simulink model "PubIfDecisionLM_MDL"  (R2020b)
settings: configuration reference "DspaceConfig" (kept outside this file)
PostLoadFcn:
  | if any(exist('dsrtsu_mdlpostloadfcn', 'file') ~= 0), dsrtsu_mdlpostloadfcn('Execute', bdroot); end
InitFcn:
  | , if any(exist('dsmpb_private', 'file') ~= 0), dsmpb_private('dsmpb_mdlclblib', 'Init', bdroot); end,
undefined symbols (not defined in the file or in its folder): OFM_OBJ_FUSIONTYPE_E, OFM_OBJ_MOVINGSTATE_E, OFM_OBJ_ORIENTATION_E, OFM_OBJ_TYPE_E, P_LM_Cyc, P_LM_EMLHistKapRcdBufSize, P_LM_EMLHistTrajBaseDis, P_LM_EMLHistTrajPNum, P_LM_EMLKapCorrMaxThre, P_LM_EMLMinKapThre, P_LM_EMLPathDisDiffThre, P_LM_EMLQuaFiltPar, P_LM_EMLTurnActKapThre, P_LM_EMLValidQuaThre, P_LM_FntPath1Disgap, P_LM_FntPath1MinDis, P_LM_FntPath1Timegap, P_LM_FntPath2Disgap, P_LM_FntPath2MinDis, P_LM_FntPath2Timegap, P_LM_FntPath3Disgap, P_LM_FntPath3MinDis, P_LM_FntPath3Timegap, P_LM_FusBLParFiltP, P_LM_FusEVDifC2Thre, P_LM_FusEVOPath1AllVSLDisThre, P_LM_FusEVOPath1AllVSLLostNumThre, P_LM_FusEVOPath1AllVSLQuaThre, P_LM_FusEVOPath1OTLFacNLC, P_LM_FusOTLQuaThre, P_LM_FusOTLSW, P_LM_FusParC0Index, P_LM_FusParC1Index, P_LM_FusParC2Index, P_LM_FusParC3Index, P_LM_FusVSLQuaThre, P_LM_FusVSLSW, P_LM_FusVSLValidSteerWheerAngThre, P_LM_FusVSLValidVxvThre, P_LM_LaneWidth, P_LM_OTLBufTPInfoEvaFactor, P_LM_OTLObjNum, P_LM_OTLObjSelectAgeThre, P_LM_OTLObjSelectDxAssessVx, P_LM_OTLObjSelectDxThre, P_LM_OTLObjSelectVxThre, P_LM_OTLObjSelectVyAssessDx, P_LM_OTLObjSelectVyThre, P_LM_OTLTrajPntBaseDis, P_LM_OTLTrajStdThre, P_LM_VSLAvailLineNum, P_LM_VSLBLSDiffThre, P_LM_VSLBLSDisRatio, P_LM_VSLFusBLParFiltP_C1, P_LM_VSLFusBLParFiltP_C2, P_LM_VSLFusBLParFiltP_C3, P_LM_VSLFusBLParFiltP_Quality, P_LM_VSLHistTrajBaseDis, P_LM_VSLHistTrajPNum, P_LM_VSLLCC0diff ... (+18)
libraries: simulink x145, LM_LIB x43
(part 20 of 24)

== matlab function PubIfDecisionLM_MDL/Subsystem2/LM_OTL/LM_OTL_MovObjTrajFit/LM_OTL_BufTPAssess/LM_OTL_BufTPInfoEva/MATLAB Function ==
  data: LM_OTLBufL1DxVect input; LM_OTLBufL2DxVect input; LM_OTLBufE1DxVect input; LM_OTLBufE2DxVect input; LM_OTLBufR1DxVect input; LM_OTLBufR2DxVect input; LM_OTLBufSPPosInfo input; LM_OTLBufEPPosInfo input; LM_OTLBufLastSPPosInfo input; LM_OTLBufLastEPPosInfo input; LM_FntPath1Dis input; LM_FntPath2Dis input; LM_FntPath3Dis input; LM_OTLBufL1LastValidInfo output; LM_OTLBufL2LastValidInfo output; LM_OTLBufE1LastValidInfo output; LM_OTLBufE2LastValidInfo output; LM_OTLBufR1LastValidInfo output; LM_OTLBufR2LastValidInfo output; LM_OTLBufL1ValidInfo output; LM_OTLBufL2ValidInfo output; LM_OTLBufE1ValidInfo output; LM_OTLBufE2ValidInfo output; LM_OTLBufR1ValidInfo output; LM_OTLBufR2ValidInfo output; P_LM_OTLBufTPInfoEvaFactor input
function [LM_OTLBufL1LastValidInfo,LM_OTLBufL2LastValidInfo,LM_OTLBufE1LastValidInfo,LM_OTLBufE2LastValidInfo,LM_OTLBufR1LastValidInfo,LM_OTLBufR2LastValidInfo,LM_OTLBufL1ValidInfo,LM_OTLBufL2ValidInfo,LM_OTLBufE1ValidInfo,LM_OTLBufE2ValidInfo,LM_OTLBufR1ValidInfo,LM_OTLBufR2ValidInfo] =fcn(LM_OTLBufL1DxVect,LM_OTLBufL2DxVect,LM_OTLBufE1DxVect,LM_OTLBufE2DxVect,LM_OTLBufR1DxVect,LM_OTLBufR2DxVect,LM_OTLBufSPPosInfo,LM_OTLBufEPPosInfo,LM_OTLBufLastSPPosInfo,LM_OTLBufLastEPPosInfo,LM_FntPath1Dis,LM_FntPath2Dis,LM_FntPath3Dis,P_LM_OTLBufTPInfoEvaFactor)

%%初始化基本参数
LM_OTLBufL1LastValidInfo=uint8(zeros(3,1));
LM_OTLBufL2LastValidInfo=uint8(zeros(3,1));
LM_OTLBufE1LastValidInfo=uint8(zeros(3,1));
LM_OTLBufE2LastValidInfo=uint8(zeros(3,1));
LM_OTLBufR1LastValidInfo=uint8(zeros(3,1));
LM_OTLBufR2LastValidInfo=uint8(zeros(3,1));
LM_OTLBufL1ValidInfo=uint8(zeros(3,1));
LM_OTLBufL2ValidInfo=uint8(zeros(3,1));
LM_OTLBufE1ValidInfo=uint8(zeros(3,1));
LM_OTLBufE2ValidInfo=uint8(zeros(3,1));
LM_OTLBufR1ValidInfo=uint8(zeros(3,1));
LM_OTLBufR2ValidInfo=uint8(zeros(3,1));
LM_FntPath0Dis=single(0);
%%计算车道线有效长度计算
FntPath1Length=LM_FntPath1Dis;
FntPath2Length=LM_FntPath2Dis-LM_FntPath1Dis;
FntPath3Length=LM_FntPath3Dis-LM_FntPath2Dis;
%%判断BufL1中前目标在各段车道线的有效值
if LM_OTLBufLastSPPosInfo(1)~=0
    %判断BufL1中前目标在前方第1段车道线的有效值
    t_buffer=[LM_OTLBufL1DxVect(LM_OTLBufLastSPPosInfo(1)),LM_OTLBufL1DxVect(LM_OTLBufLastEPPosInfo(1)),LM_FntPath0Dis,LM_FntPath1Dis];
    t_LMlength=abs(LM_OTLBufL1DxVect(LM_OTLBufLastSPPosInfo(1))-LM_OTLBufL1DxVect(LM_OTLBufLastEPPosInfo(1)));
    t_length=max(t_buffer)-min(t_buffer);
    t_overlap=FntPath1Length+t_LMlength-t_length;
    if t_overlap<P_LM_OTLBufTPInfoEvaFactor*FntPath1Length
        LM_OTLBufL1LastFntPath1Valid=0;
    else
        LM_OTLBufL1LastFntPath1Valid=1;
    end
    %判断BufL1中前目标在前方第2段车道线的有效值
    t_buffer=[LM_OTLBufL1DxVect(LM_OTLBufLastSPPosInfo(1)),LM_OTLBufL1DxVect(LM_OTLBufLastEPPosInfo(1)),LM_FntPath2Dis,LM_FntPath1Dis];
    t_length=max(t_buffer)-min(t_buffer);
    t_overlap=FntPath2Length+t_LMlength-t_length;
    if t_overlap<P_LM_OTLBufTPInfoEvaFactor*FntPath2Length
        LM_OTLBufL1LastFntPath2Valid=0;
    else
        LM_OTLBufL1LastFntPath2Valid=1;
    end
    %判断BufL1中前目标在前方第3段车道线的有效值
    t_buffer=[LM_OTLBufL1DxVect(LM_OTLBufLastSPPosInfo(1)),LM_OTLBufL1DxVect(LM_OTLBufLastEPPosInfo(1)),LM_FntPath2Dis,LM_FntPath3Dis];
    t_length=max(t_buffer)-min(t_buffer);
    t_overlap=FntPath3Length+t_LMlength-t_length;
    if t_overlap<P_LM_OTLBufTPInfoEvaFactor*FntPath3Length
        LM_OTLBufL1LastFntPath3Valid=0;
    else
        LM_OTLBufL1LastFntPath3Valid=1;
    end 
else
    LM_OTLBufL1LastFntPath1Valid=0;
    LM_OTLBufL1LastFntPath2Valid=0;
    LM_OTLBufL1LastFntPath3Valid=0;
end
LM_OTLBufL1LastValidInfo(1)=LM_OTLBufL1LastFntPath1Valid;
LM_OTLBufL1LastValidInfo(2)=LM_OTLBufL1LastFntPath2Valid;
LM_OTLBufL1LastValidInfo(3)=LM_OTLBufL1LastFntPath3Valid;
%%判断BufL1当前目标在各段车道线的有效值
if LM_OTLBufSPPosInfo(1)~=0
    %判断BufL1当前目标在前方第1段车道线的有效值
    t_LMlength=abs(LM_OTLBufL1DxVect(LM_OTLBufSPPosInfo(1))-LM_OTLBufL1DxVect(LM_OTLBufEPPosInfo(1)));
    t_buffer=[LM_OTLBufL1DxVect(LM_OTLBufSPPosInfo(1)),LM_OTLBufL1DxVect(LM_OTLBufEPPosInfo(1)),LM_FntPath0Dis,LM_FntPath1Dis];
    t_length=max(t_buffer)-min(t_buffer);
    t_overlap=FntPath1Length+t_LMlength-t_length;
    if t_overlap<P_LM_OTLBufTPInfoEvaFactor*FntPath1Length
        LM_OTLBufL1FntPath1Valid=0;
    else
        LM_OTLBufL1FntPath1Valid=1;
    end
    %判断BufL1当前目标在前方第2段车道线的有效值
    t_buffer=[LM_OTLBufL1DxVect(LM_OTLBufSPPosInfo(1)),LM_OTLBufL1DxVect(LM_OTLBufEPPosInfo(1)),LM_FntPath2Dis,LM_FntPath1Dis];
    t_length=max(t_buffer)-min(t_buffer);
    t_overlap=FntPath2Length+t_LMlength-t_length;
    if t_overlap<P_LM_OTLBufTPInfoEvaFactor*FntPath2Length
        LM_OTLBufL1FntPath2Valid=0;
    else
        LM_OTLBufL1FntPath2Valid=1;
    end
    %判断BufL1当前目标在前方第3段车道线的有效值
    t_buffer=[LM_OTLBufL1DxVect(LM_OTLBufSPPosInfo(1)),LM_OTLBufL1DxVect(LM_OTLBufEPPosInfo(1)),LM_FntPath2Dis,LM_FntPath3Dis];
    t_length=max(t_buffer)-min(t_buffer);
    t_overlap=FntPath3Length+t_LMlength-t_length;
    if t_overlap<P_LM_OTLBufTPInfoEvaFactor*FntPath3Length
        LM_OTLBufL1FntPath3Valid=0;
    else
        LM_OTLBufL1FntPath3Valid=1;
    end 
else
    LM_OTLBufL1FntPath1Valid=0;
    LM_OTLBufL1FntPath2Valid=0;
    LM_OTLBufL1FntPath3Valid=0;
end
LM_OTLBufL1ValidInfo(1)=LM_OTLBufL1FntPath1Valid;
LM_OTLBufL1ValidInfo(2)=LM_OTLBufL1FntPath2Valid;
LM_OTLBufL1ValidInfo(3)=LM_OTLBufL1FntPath3Valid;
%%判断BufL2中前目标在各段车道线的有效值
if LM_OTLBufLastSPPosInfo(2)~=0
    %判断BufL2中前目标在前方第1段车道线的有效值
    t_LMlength=abs(LM_OTLBufL2DxVect(LM_OTLBufLastSPPosInfo(2))-LM_OTLBufL2DxVect(LM_OTLBufLastEPPosInfo(2)));
    t_buffer=[LM_OTLBufL2DxVect(LM_OTLBufLastSPPosInfo(2)),LM_OTLBufL2DxVect(LM_OTLBufLastEPPosInfo(2)),LM_FntPath0Dis,LM_FntPath1Dis];
    t_length=max(t_buffer)-min(t_buffer);
    t_overlap=FntPath1Length+t_LMlength-t_length;
    if t_overlap<P_LM_OTLBufTPInfoEvaFactor*FntPath1Length
        LM_OTLBufL2LastFntPath1Valid=0;
    else
        LM_OTLBufL2LastFntPath1Valid=1;
    end
    %判断BufL2中前目标在前方第2段车道线的有效值
    t_buffer=[LM_OTLBufL2DxVect(LM_OTLBufLastSPPosInfo(2)),LM_OTLBufL2DxVect(LM_OTLBufLastEPPosInfo(2)),LM_FntPath2Dis,LM_FntPath1Dis];
    t_length=max(t_buffer)-min(t_buffer);
    t_overlap=FntPath2Length+t_LMlength-t_length;
    if t_overlap<P_LM_OTLBufTPInfoEvaFactor*FntPath2Length
        LM_OTLBufL2LastFntPath2Valid=0;
    else
        LM_OTLBufL2LastFntPath2Valid=1;
    end
    %判断BufL2中前目标在前方第3段车道线的有效值
    t_buffer=[LM_OTLBufL2DxVect(LM_OTLBufLastSPPosInfo(2)),LM_OTLBufL2DxVect(LM_OTLBufLastEPPosInfo(2)),LM_FntPath2Dis,LM_FntPath3Dis];
    t_length=max(t_buffer)-min(t_buffer);
    t_overlap=FntPath3Length+t_LMlength-t_length;
    if t_overlap<P_LM_OTLBufTPInfoEvaFactor*FntPath3Length
        LM_OTLBufL2LastFntPath3Valid=0;
    else
        LM_OTLBufL2LastFntPath3Valid=1;
    end 
else
    LM_OTLBufL2LastFntPath1Valid=0;
    LM_OTLBufL2LastFntPath2Valid=0;
    LM_OTLBufL2LastFntPath3Valid=0;
end
LM_OTLBufL2LastValidInfo(1)=LM_OTLBufL2LastFntPath1Valid;
LM_OTLBufL2LastValidInfo(2)=LM_OTLBufL2LastFntPath2Valid;
LM_OTLBufL2LastValidInfo(3)=LM_OTLBufL2LastFntPath3Valid;
%%判断BufL2当前目标在各段车道线的有效值
if LM_OTLBufSPPosInfo(2)~=0
    %判断BufL2当前目标在前方第1段车道线的有效值
    t_LMlength=abs(LM_OTLBufL2DxVect(LM_OTLBufSPPosInfo(2))-LM_OTLBufL2DxVect(LM_OTLBufEPPosInfo(2)));
    t_buffer=[LM_OTLBufL2DxVect(LM_OTLBufSPPosInfo(2)),LM_OTLBufL2DxVect(LM_OTLBufEPPosInfo(2)),LM_FntPath0Dis,LM_FntPath1Dis];
    t_length=max(t_buffer)-min(t_buffer);
    t_overlap=FntPath1Length+t_LMlength-t_length;
    if t_overlap<P_LM_OTLBufTPInfoEvaFactor*FntPath1Length
        LM_OTLBufL2FntPath1Valid=0;
    else
        LM_OTLBufL2FntPath1Valid=1;
    end
    %判断BufL2当前目标在前方第2段车道线的有效值
    t_buffer=[LM_OTLBufL2DxVect(LM_OTLBufSPPosInfo(2)),LM_OTLBufL2DxVect(LM_OTLBufEPPosInfo(2)),LM_FntPath2Dis,LM_FntPath1Dis];
    t_length=max(t_buffer)-min(t_buffer);
    t_overlap=FntPath2Length+t_LMlength-t_length;
    if t_overlap<P_LM_OTLBufTPInfoEvaFactor*FntPath2Length
        LM_OTLBufL2FntPath2Valid=0;
    else
        LM_OTLBufL2FntPath2Valid=1;
    end
    %判断BufL2当前目标在前方第3段车道线的有效值
    t_buffer=[LM_OTLBufL2DxVect(LM_OTLBufSPPosInfo(2)),LM_OTLBufL2DxVect(LM_OTLBufEPPosInfo(2)),LM_FntPath2Dis,LM_FntPath3Dis];
    t_length=max(t_buffer)-min(t_buffer);
    t_overlap=FntPath3Length+t_LMlength-t_length;
    if t_overlap<P_LM_OTLBufTPInfoEvaFactor*FntPath3Length
        LM_OTLBufL2FntPath3Valid=0;
    else
        LM_OTLBufL2FntPath3Valid=1;
    end 
else
    LM_OTLBufL2FntPath1Valid=0;
    LM_OTLBufL2FntPath2Valid=0;
    LM_OTLBufL2FntPath3Valid=0;
end
LM_OTLBufL2ValidInfo(1)=LM_OTLBufL2FntPath1Valid;
LM_OTLBufL2ValidInfo(2)=LM_OTLBufL2FntPath2Valid;
LM_OTLBufL2ValidInfo(3)=LM_OTLBufL2FntPath3Valid;
%%判断BufE1中前目标在各段车道线的有效值
if LM_OTLBufLastSPPosInfo(3)~=0
    %判断BufE1中前目标在前方第1段车道线的有效值
    t_LMlength=abs(LM_OTLBufE1DxVect(LM_OTLBufLastSPPosInfo(3))-LM_OTLBufE1DxVect(LM_OTLBufLastEPPosInfo(3)));
    t_buffer=[LM_OTLBufE1DxVect(LM_OTLBufLastSPPosInfo(3)),LM_OTLBufE1DxVect(LM_OTLBufLastEPPosInfo(3)),LM_FntPath0Dis,LM_FntPath1Dis];
    t_length=max(t_buffer)-min(t_buffer);
    t_overlap=FntPath1Length+t_LMlength-t_length;
    if t_overlap<P_LM_OTLBufTPInfoEvaFactor*FntPath1Length
        LM_OTLBufE1LastFntPath1Valid=0;
    else
        LM_OTLBufE1LastFntPath1Valid=1;
    end
    %判断BufE1中前目标在前方第2段车道线的有效值
    t_buffer=[LM_OTLBufE1DxVect(LM_OTLBufLastSPPosInfo(3)),LM_OTLBufE1DxVect(LM_OTLBufLastEPPosInfo(3)),LM_FntPath2Dis,LM_FntPath1Dis];
    t_length=max(t_buffer)-min(t_buffer);
    t_overlap=FntPath2Length+t_LMlength-t_length;
    if t_overlap<P_LM_OTLBufTPInfoEvaFactor*FntPath2Length
        LM_OTLBufE1LastFntPath2Valid=0;
    else
        LM_OTLBufE1LastFntPath2Valid=1;
    end
    %判断BufE1中前目标在前方第3段车道线的有效值
    t_buffer=[LM_OTLBufE1DxVect(LM_OTLBufLastSPPosInfo(3)),LM_OTLBufE1DxVect(LM_OTLBufLastEPPosInfo(3)),LM_FntPath2Dis,LM_FntPath3Dis];
    t_length=max(t_buffer)-min(t_buffer);
    t_overlap=FntPath3Length+t_LMlength-t_length;
    if t_overlap<P_LM_OTLBufTPInfoEvaFactor*FntPath3Length
        LM_OTLBufE1LastFntPath3Valid=0;
    else
        LM_OTLBufE1LastFntPath3Valid=1;
    end 
else
    LM_OTLBufE1LastFntPath1Valid=0;
    LM_OTLBufE1LastFntPath2Valid=0;
    LM_OTLBufE1LastFntPath3Valid=0;
end
LM_OTLBufE1LastValidInfo(1)=LM_OTLBufE1LastFntPath1Valid;
LM_OTLBufE1LastValidInfo(2)=LM_OTLBufE1LastFntPath2Valid;
LM_OTLBufE1LastValidInfo(3)=LM_OTLBufE1LastFntPath3Valid;
%%判断BufE1当前目标在各段车道线的有效值
if LM_OTLBufSPPosInfo(3)~=0
    %判断BufE1当前目标在前方第1段车道线的有效值
    t_LMlength=abs(LM_OTLBufE1DxVect(LM_OTLBufSPPosInfo(3))-LM_OTLBufE1DxVect(LM_OTLBufEPPosInfo(3)));
    t_buffer=[LM_OTLBufE1DxVect(LM_OTLBufSPPosInfo(3)),LM_OTLBufE1DxVect(LM_OTLBufEPPosInfo(3)),LM_FntPath0Dis,LM_FntPath1Dis];
    t_length=max(t_buffer)-min(t_buffer);
    t_overlap=FntPath1Length+t_LMlength-t_length;
    if t_overlap<P_LM_OTLBufTPInfoEvaFactor*FntPath1Length
        LM_OTLBufE1FntPath1Valid=0;
    else
        LM_OTLBufE1FntPath1Valid=1;
    end
    %判断BufE1当前目标在前方第2段车道线的有效值
    t_buffer=[LM_OTLBufE1DxVect(LM_OTLBufSPPosInfo(3)),LM_OTLBufE1DxVect(LM_OTLBufEPPosInfo(3)),LM_FntPath2Dis,LM_FntPath1Dis];
    t_length=max(t_buffer)-min(t_buffer);
    t_overlap=FntPath2Length+t_LMlength-t_length;
    if t_overlap<P_LM_OTLBufTPInfoEvaFactor*FntPath2Length
        LM_OTLBufE1FntPath2Valid=0;
    else
        LM_OTLBufE1FntPath2Valid=1;
    end
    %判断BufE1当前目标在前方第3段车道线的有效值
    t_buffer=[LM_OTLBufE1DxVect(LM_OTLBufSPPosInfo(3)),LM_OTLBufE1DxVect(LM_OTLBufEPPosInfo(3)),LM_FntPath2Dis,LM_FntPath3Dis];
    t_length=max(t_buffer)-min(t_buffer);
    t_overlap=FntPath3Length+t_LMlength-t_length;
    if t_overlap<P_LM_OTLBufTPInfoEvaFactor*FntPath3Length
        LM_OTLBufE1FntPath3Valid=0;
    else
        LM_OTLBufE1FntPath3Valid=1;
    end 
else
    LM_OTLBufE1FntPath1Valid=0;
    LM_OTLBufE1FntPath2Valid=0;
    LM_OTLBufE1FntPath3Valid=0;
end
LM_OTLBufE1ValidInfo(1)=LM_OTLBufE1FntPath1Valid;
LM_OTLBufE1ValidInfo(2)=LM_OTLBufE1FntPath2Valid;
LM_OTLBufE1ValidInfo(3)=LM_OTLBufE1FntPath3Valid;
%%判断BufE2中前目标在各段车道线的有效值
if LM_OTLBufLastSPPosInfo(4)~=0
    %判断BufE2中前目标在前方第1段车道线的有效值
    t_LMlength=abs(LM_OTLBufE2DxVect(LM_OTLBufLastSPPosInfo(4))-LM_OTLBufE2DxVect(LM_OTLBufLastEPPosInfo(4)));
    t_buffer=[LM_OTLBufE2DxVect(LM_OTLBufLastSPPosInfo(4)),LM_OTLBufE2DxVect(LM_OTLBufLastEPPosInfo(4)),LM_FntPath0Dis,LM_FntPath1Dis];
    t_length=max(t_buffer)-min(t_buffer);
    t_overlap=FntPath1Length+t_LMlength-t_length;
    if t_overlap<P_LM_OTLBufTPInfoEvaFactor*FntPath1Length
        LM_OTLBufE2LastFntPath1Valid=0;
    else
        LM_OTLBufE2LastFntPath1Valid=1;
    end
    %判断BufE2中前目标在前方第2段车道线的有效值
    t_buffer=[LM_OTLBufE2DxVect(LM_OTLBufLastSPPosInfo(4)),LM_OTLBufE2DxVect(LM_OTLBufLastEPPosInfo(4)),LM_FntPath2Dis,LM_FntPath1Dis];
    t_length=max(t_buffer)-min(t_buffer);
    t_overlap=FntPath2Length+t_LMlength-t_length;
    if t_overlap<P_LM_OTLBufTPInfoEvaFactor*FntPath2Length
        LM_OTLBufE2LastFntPath2Valid=0;
    else
        LM_OTLBufE2LastFntPath2Valid=1;
    end
    %判断BufE2中前目标在前方第3段车道线的有效值
    t_buffer=[LM_OTLBufE2DxVect(LM_OTLBufLastSPPosInfo(4)),LM_OTLBufE2DxVect(LM_OTLBufLastEPPosInfo(4)),LM_FntPath2Dis,LM_FntPath3Dis];
    t_length=max(t_buffer)-min(t_buffer);
    t_overlap=FntPath3Length+t_LMlength-t_length;
    if t_overlap<P_LM_OTLBufTPInfoEvaFactor*FntPath3Length
        LM_OTLBufE2LastFntPath3Valid=0;
    else
        LM_OTLBufE2LastFntPath3Valid=1;
    end 
else
    LM_OTLBufE2LastFntPath1Valid=0;
    LM_OTLBufE2LastFntPath2Valid=0;
    LM_OTLBufE2LastFntPath3Valid=0;
end
LM_OTLBufE2LastValidInfo(1)=LM_OTLBufE2LastFntPath1Valid;
LM_OTLBufE2LastValidInfo(2)=LM_OTLBufE2LastFntPath2Valid;
LM_OTLBufE2LastValidInfo(3)=LM_OTLBufE2LastFntPath3Valid;
%%判断BufE2当前目标在各段车道线的有效值
if LM_OTLBufSPPosInfo(4)~=0
    %判断BufE2当前目标在前方第1段车道线的有效值
    t_LMlength=abs(LM_OTLBufE2DxVect(LM_OTLBufSPPosInfo(4))-LM_OTLBufE2DxVect(LM_OTLBufEPPosInfo(4)));
    t_buffer=[LM_OTLBufE2DxVect(LM_OTLBufSPPosInfo(4)),LM_OTLBufE2DxVect(LM_OTLBufEPPosInfo(4)),LM_FntPath0Dis,LM_FntPath1Dis];
    t_length=max(t_buffer)-min(t_buffer);
    t_overlap=FntPath1Length+t_LMlength-t_length;
    if t_overlap<P_LM_OTLBufTPInfoEvaFactor*FntPath1Length
        LM_OTLBufE2FntPath1Valid=0;
    else
        LM_OTLBufE2FntPath1Valid=1;
    end
    %判断BufE2当前目标在前方第2段车道线的有效值
    t_buffer=[LM_OTLBufE2DxVect(LM_OTLBufSPPosInfo(4)),LM_OTLBufE2DxVect(LM_OTLBufEPPosInfo(4)),LM_FntPath2Dis,LM_FntPath1Dis];
    t_length=max(t_buffer)-min(t_buffer);
    t_overlap=FntPath2Length+t_LMlength-t_length;
    if t_overlap<P_LM_OTLBufTPInfoEvaFactor*FntPath2Length
        LM_OTLBufE2FntPath2Valid=0;
    else
        LM_OTLBufE2FntPath2Valid=1;
    end
    %判断BufE2当前目标在前方第3段车道线的有效值
    t_buffer=[LM_OTLBufE2DxVect(LM_OTLBufSPPosInfo(4)),LM_OTLBufE2DxVect(LM_OTLBufEPPosInfo(4)),LM_FntPath2Dis,LM_FntPath3Dis];
    t_length=max(t_buffer)-min(t_buffer);
    t_overlap=FntPath3Length+t_LMlength-t_length;
    if t_overlap<P_LM_OTLBufTPInfoEvaFactor*FntPath3Length
        LM_OTLBufE2FntPath3Valid=0;
    else
        LM_OTLBufE2FntPath3Valid=1;
    end 
else
    LM_OTLBufE2FntPath1Valid=0;
    LM_OTLBufE2FntPath2Valid=0;
    LM_OTLBufE2FntPath3Valid=0;
end
LM_OTLBufE2ValidInfo(1)=LM_OTLBufE2FntPath1Valid;
LM_OTLBufE2ValidInfo(2)=LM_OTLBufE2FntPath2Valid;
LM_OTLBufE2ValidInfo(3)=LM_OTLBufE2FntPath3Valid;
%%判断BufR1中前目标在各段车道线的有效值
if LM_OTLBufLastSPPosInfo(5)~=0
    %判断BufR1中前目标在前方第1段车道线的有效值
    t_LMlength=abs(LM_OTLBufR1DxVect(LM_OTLBufLastSPPosInfo(5))-LM_OTLBufR1DxVect(LM_OTLBufLastEPPosInfo(5)));
    t_buffer=[LM_OTLBufR1DxVect(LM_OTLBufLastSPPosInfo(5)),LM_OTLBufR1DxVect(LM_OTLBufLastEPPosInfo(5)),LM_FntPath0Dis,LM_FntPath1Dis];
    t_length=max(t_buffer)-min(t_buffer);
    t_overlap=FntPath1Length+t_LMlength-t_length;
    if t_overlap<P_LM_OTLBufTPInfoEvaFactor*FntPath1Length
        LM_OTLBufR1LastFntPath1Valid=0;
    else
        LM_OTLBufR1LastFntPath1Valid=1;
    end
    %判断BufR1中前目标在前方第2段车道线的有效值
    t_buffer=[LM_OTLBufR1DxVect(LM_OTLBufLastSPPosInfo(5)),LM_OTLBufR1DxVect(LM_OTLBufLastEPPosInfo(5)),LM_FntPath2Dis,LM_FntPath1Dis];
    t_length=max(t_buffer)-min(t_buffer);
    t_overlap=FntPath2Length+t_LMlength-t_length;
    if t_overlap<P_LM_OTLBufTPInfoEvaFactor*FntPath2Length
        LM_OTLBufR1LastFntPath2Valid=0;
    else
        LM_OTLBufR1LastFntPath2Valid=1;
    end
    %判断BufR1中前目标在前方第3段车道线的有效值
    t_buffer=[LM_OTLBufR1DxVect(LM_OTLBufLastSPPosInfo(5)),LM_OTLBufR1DxVect(LM_OTLBufLastEPPosInfo(5)),LM_FntPath2Dis,LM_FntPath3Dis];
    t_length=max(t_buffer)-min(t_buffer);
    t_overlap=FntPath3Length+t_LMlength-t_length;
    if t_overlap<P_LM_OTLBufTPInfoEvaFactor*FntPath3Length
        LM_OTLBufR1LastFntPath3Valid=0;
    else
        LM_OTLBufR1LastFntPath3Valid=1;
    end 
else
    LM_OTLBufR1LastFntPath1Valid=0;
    LM_OTLBufR1LastFntPath2Valid=0;
    LM_OTLBufR1LastFntPath3Valid=0;
end
LM_OTLBufR1LastValidInfo(1)=LM_OTLBufR1LastFntPath1Valid;
LM_OTLBufR1LastValidInfo(2)=LM_OTLBufR1LastFntPath2Valid;
LM_OTLBufR1LastValidInfo(3)=LM_OTLBufR1LastFntPath3Valid;
%%判断BufR1当前目标在各段车道线的有效值
if LM_OTLBufSPPosInfo(5)~=0
    %判断BufR1当前目标在前方第1段车道线的有效值
    t_LMlength=abs(LM_OTLBufR1DxVect(LM_OTLBufSPPosInfo(5))-LM_OTLBufR1DxVect(LM_OTLBufEPPosInfo(5)));
    t_buffer=[LM_OTLBufR1DxVect(LM_OTLBufSPPosInfo(5)),LM_OTLBufR1DxVect(LM_OTLBufEPPosInfo(5)),LM_FntPath0Dis,LM_FntPath1Dis];
    t_length=max(t_buffer)-min(t_buffer);
    t_overlap=FntPath1Length+t_LMlength-t_length;
    if t_overlap<P_LM_OTLBufTPInfoEvaFactor*FntPath1Length
        LM_OTLBufR1FntPath1Valid=0;
    else
        LM_OTLBufR1FntPath1Valid=1;
    end
    %判断BufR1当前目标在前方第2段车道线的有效值
    t_buffer=[LM_OTLBufR1DxVect(LM_OTLBufSPPosInfo(5)),LM_OTLBufR1DxVect(LM_OTLBufEPPosInfo(5)),LM_FntPath2Dis,LM_FntPath1Dis];
    t_length=max(t_buffer)-min(t_buffer);
    t_overlap=FntPath2Length+t_LMlength-t_length;
    if t_overlap<P_LM_OTLBufTPInfoEvaFactor*FntPath2Length
        LM_OTLBufR1FntPath2Valid=0;
    else
        LM_OTLBufR1FntPath2Valid=1;
    end
    %判断BufR1当前目标在前方第3段车道线的有效值
    t_buffer=[LM_OTLBufR1DxVect(LM_OTLBufSPPosInfo(5)),LM_OTLBufR1DxVect(LM_OTLBufEPPosInfo(5)),LM_FntPath2Dis,LM_FntPath3Dis];
    t_length=max(t_buffer)-min(t_buffer);
    t_overlap=FntPath3Length+t_LMlength-t_length;
    if t_overlap<P_LM_OTLBufTPInfoEvaFactor*FntPath3Length
        LM_OTLBufR1FntPath3Valid=0;
    else
        LM_OTLBufR1FntPath3Valid=1;
    end 
else
    LM_OTLBufR1FntPath1Valid=0;
    LM_OTLBufR1FntPath2Valid=0;
    LM_OTLBufR1FntPath3Valid=0;
end
LM_OTLBufR1ValidInfo(1)=LM_OTLBufR1FntPath1Valid;
LM_OTLBufR1ValidInfo(2)=LM_OTLBufR1FntPath2Valid;
LM_OTLBufR1ValidInfo(3)=LM_OTLBufR1FntPath3Valid;
%%判断BufR2中前目标在各段车道线的有效值
if LM_OTLBufLastSPPosInfo(6)~=0
    %判断BufR2中前目标在前方第1段车道线的有效值
    t_LMlength=abs(LM_OTLBufR2DxVect(LM_OTLBufLastSPPosInfo(6))-LM_OTLBufR2DxVect(LM_OTLBufLastEPPosInfo(6)));
    t_buffer=[LM_OTLBufR2DxVect(LM_OTLBufLastSPPosInfo(6)),LM_OTLBufR2DxVect(LM_OTLBufLastEPPosInfo(6)),LM_FntPath0Dis,LM_FntPath1Dis];
    t_length=max(t_buffer)-min(t_buffer);
    t_overlap=FntPath1Length+t_LMlength-t_length;
    if t_overlap<P_LM_OTLBufTPInfoEvaFactor*FntPath1Length
        LM_OTLBufR2LastFntPath1Valid=0;
    else
        LM_OTLBufR2LastFntPath1Valid=1;
    end
    %判断BufR2中前目标在前方第2段车道线的有效值
    t_buffer=[LM_OTLBufR2DxVect(LM_OTLBufLastSPPosInfo(6)),LM_OTLBufR2DxVect(LM_OTLBufLastEPPosInfo(6)),LM_FntPath2Dis,LM_FntPath1Dis];
    t_length=max(t_buffer)-min(t_buffer);
    t_overlap=FntPath2Length+t_LMlength-t_length;
    if t_overlap<P_LM_OTLBufTPInfoEvaFactor*FntPath2Length
        LM_OTLBufR2LastFntPath2Valid=0;
    else
        LM_OTLBufR2LastFntPath2Valid=1;
    end
    %判断BufR2中前目标在前方第3段车道线的有效值
    t_buffer=[LM_OTLBufR2DxVect(LM_OTLBufLastSPPosInfo(6)),LM_OTLBufR2DxVect(LM_OTLBufLastEPPosInfo(6)),LM_FntPath2Dis,LM_FntPath3Dis];
    t_length=max(t_buffer)-min(t_buffer);
    t_overlap=FntPath3Length+t_LMlength-t_length;
    if t_overlap<P_LM_OTLBufTPInfoEvaFactor*FntPath3Length
        LM_OTLBufR2LastFntPath3Valid=0;
    else
        LM_OTLBufR2LastFntPath3Valid=1;
    end 
else
    LM_OTLBufR2LastFntPath1Valid=0;
    LM_OTLBufR2LastFntPath2Valid=0;
    LM_OTLBufR2LastFntPath3Valid=0;
end
LM_OTLBufR2LastValidInfo(1)=LM_OTLBufR2LastFntPath1Valid;
LM_OTLBufR2LastValidInfo(2)=LM_OTLBufR2LastFntPath2Valid;
LM_OTLBufR2LastValidInfo(3)=LM_OTLBufR2LastFntPath3Valid;
%%判断BufR2当前目标在各段车道线的有效值
if LM_OTLBufSPPosInfo(6)~=0
    %判断BufR2当前目标在前方第1段车道线的有效值
    t_LMlength=abs(LM_OTLBufR2DxVect(LM_OTLBufSPPosInfo(6))-LM_OTLBufR2DxVect(LM_OTLBufEPPosInfo(6)));
    t_buffer=[LM_OTLBufR2DxVect(LM_OTLBufSPPosInfo(6)),LM_OTLBufR2DxVect(LM_OTLBufEPPosInfo(6)),LM_FntPath0Dis,LM_FntPath1Dis];
    t_length=max(t_buffer)-min(t_buffer);
    t_overlap=FntPath1Length+t_LMlength-t_length;
    if t_overlap<P_LM_OTLBufTPInfoEvaFactor*FntPath1Length
        LM_OTLBufR2FntPath1Valid=0;
    else
        LM_OTLBufR2FntPath1Valid=1;
    end
    %判断BufR2当前目标在前方第2段车道线的有效值
    t_buffer=[LM_OTLBufR2DxVect(LM_OTLBufSPPosInfo(6)),LM_OTLBufR2DxVect(LM_OTLBufEPPosInfo(6)),LM_FntPath2Dis,LM_FntPath1Dis];
    t_length=max(t_buffer)-min(t_buffer);
    t_overlap=FntPath2Length+t_LMlength-t_length;
    if t_overlap<P_LM_OTLBufTPInfoEvaFactor*FntPath2Length
        LM_OTLBufR2FntPath2Valid=0;
    else
        LM_OTLBufR2FntPath2Valid=1;
    end
    %判断BufR2当前目标在前方第3段车道线的有效值
    t_buffer=[LM_OTLBufR2DxVect(LM_OTLBufSPPosInfo(6)),LM_OTLBufR2DxVect(LM_OTLBufEPPosInfo(6)),LM_FntPath2Dis,LM_FntPath3Dis];
    t_length=max(t_buffer)-min(t_buffer);
    t_overlap=FntPath3Length+t_LMlength-t_length;
    if t_overlap<P_LM_OTLBufTPInfoEvaFactor*FntPath3Length
        LM_OTLBufR2FntPath3Valid=0;
    else
        LM_OTLBufR2FntPath3Valid=1;
    end 
else
    LM_OTLBufR2FntPath1Valid=0;
    LM_OTLBufR2FntPath2Valid=0;
    LM_OTLBufR2FntPath3Valid=0;
end
LM_OTLBufR2ValidInfo(1)=LM_OTLBufR2FntPath1Valid;
LM_OTLBufR2ValidInfo(2)=LM_OTLBufR2FntPath2Valid;
LM_OTLBufR2ValidInfo(3)=LM_OTLBufR2FntPath3Valid;
end

== matlab function PubIfDecisionLM_MDL/Subsystem2/LM_OTL/LM_OTL_MovObjTrajFit/LM_OTL_BufTPAssess/LM_OTL_BufTrajEva/Subsystem/MATLAB Function1 ==
  data: Offset output; Flg output; LM_OTLBufValidInfo input; LM_OTLDxVect input; LM_OTLDyVect input; LM_OTLSPPos input; LM_OTLEPPos input; LM_FntPath1Dis input; LM_FntPath2Dis input; LM_FntPath3Dis input; TpValidNum output; SPValidPos output; P_LM_OTLTrajStdThre input
function [Offset,Flg,TpValidNum,SPValidPos] = fcn(LM_OTLBufValidInfo,LM_OTLDxVect,LM_OTLDyVect,LM_OTLSPPos,LM_OTLEPPos,LM_FntPath1Dis,LM_FntPath2Dis,LM_FntPath3Dis, P_LM_OTLTrajStdThre)


%%第一段前车道线取点
Offset=single(zeros(3,1));
Flg=uint8(zeros(3,1));
TpValidNum=uint8(zeros(3,1));
SPValidPos=uint8(zeros(3,1));
t_pnum=uint8(0);
t_sumy=single(0);
t_sumerry=single(0);
t_index=uint8(0);
if LM_OTLBufValidInfo(1)~=0
    if LM_OTLEPPos>=LM_OTLSPPos
        for i=LM_OTLSPPos:LM_OTLEPPos
            if LM_OTLDxVect(i)>0&&LM_OTLDxVect(i)<=LM_FntPath1Dis
                t_pnum=t_pnum+uint8(1);
                t_index=i;
                t_sumy=t_sumy+LM_OTLDyVect(i);
            end
        end
        t_mean=t_sumy/single(t_pnum);
        SPValidPos(1)=t_index-t_pnum+uint8(1);
        for i=t_index:-1:SPValidPos(1)
            t_error=(LM_OTLDyVect(i)-t_mean)^2;
            t_sumerry=t_sumerry+t_error;
        end
        if sqrt(t_sumerry/single(t_pnum))<=P_LM_OTLTrajStdThre
           Offset(1)=t_mean;
           Flg(1)=uint8(1);
           TpValidNum(1)=t_pnum;
        end
    elseif LM_OTLEPPos<LM_OTLSPPos
        for i=LM_OTLSPPos:80
            if LM_OTLDxVect(i)>0&&LM_OTLDxVect(i)<=LM_FntPath1Dis
                t_pnum=t_pnum+uint8(1);
                t_index=i;
                t_sumy=t_sumy+LM_OTLDyVect(i);
            end
        end
        for i=1:LM_OTLEPPos 
            if LM_OTLDxVect(i)>0&&LM_OTLDxVect(i)<=LM_FntPath1Dis
                t_pnum=t_pnum+uint8(1);
                t_index=i;
                t_sumy=t_sumy+LM_OTLDyVect(i);
            end
        end
        SPValidPos(1)=uint8(81)+t_index-t_pnum;
        t_mean=t_sumy/single(t_pnum);
        if SPValidPos(1)>80
            SPValidPos(1)=SPValidPos(1)-80;
        end
        if (SPValidPos(1)>=LM_OTLSPPos&&t_index>=LM_OTLSPPos)||(SPValidPos(1)<LM_OTLSPPos&&t_index<LM_OTLSPPos)
            for i=t_index:-1:SPValidPos(1)
                t_error=(LM_OTLDyVect(i)-t_mean)^2;
                t_sumerry=t_sumerry+t_error;
            end
        else
            for i=1:t_index
                t_error=(LM_OTLDyVect(i)-t_mean)^2;
                t_sumerry=t_sumerry+t_error;
            end
            for i=80:-1:SPValidPos(1)
                 t_error=(LM_OTLDyVect(i)-t_mean)^2;
                t_sumerry=t_sumerry+t_error;
            end
        end
        if sqrt(t_sumerry/single(t_pnum))<=P_LM_OTLTrajStdThre
           Offset(1)=t_mean;
           Flg(1)=uint8(1);
           TpValidNum(1)=t_pnum;
        end           
    end
end
%%第二段前车道线取点
t_pnum=uint8(0);
t_sumy=single(0);
t_sumerry=single(0);
t_index=uint8(0);
if LM_OTLBufValidInfo(2)~=0
    if LM_OTLEPPos>=LM_OTLSPPos
        for i=LM_OTLSPPos:LM_OTLEPPos
            if LM_OTLDxVect(i)>LM_FntPath1Dis&&LM_OTLDxVect(i)<=LM_FntPath2Dis
                t_pnum=t_pnum+uint8(1);
                t_index=i;
                t_sumy=t_sumy+LM_OTLDyVect(i);
            end
        end
        t_mean=t_sumy/single(t_pnum);
        SPValidPos(2)=t_index-t_pnum+uint8(1);
        for i=t_index:-1:SPValidPos(2)
            t_error=(LM_OTLDyVect(i)-t_mean)^2;
            t_sumerry=t_sumerry+t_error;
        end
        if sqrt(t_sumerry/single(t_pnum))<=P_LM_OTLTrajStdThre
           Offset(2)=t_mean;
           Flg(2)=uint8(1);
           TpValidNum(2)=t_pnum;
        end
    elseif LM_OTLEPPos<LM_OTLSPPos
        for i=LM_OTLSPPos:80
            if LM_OTLDxVect(i)>LM_FntPath1Dis&&LM_OTLDxVect(i)<=LM_FntPath2Dis
                t_pnum=t_pnum+uint8(1);
                t_index=i;
                t_sumy=t_sumy+LM_OTLDyVect(i);
            end
        end
        for i=1:LM_OTLEPPos 
            if LM_OTLDxVect(i)>LM_FntPath1Dis&&LM_OTLDxVect(i)<=LM_FntPath2Dis
                t_pnum=t_pnum+uint8(1);
                t_index=i;
                t_sumy=t_sumy+LM_OTLDyVect(i);
            end
        end
        t_mean=t_sumy/single(t_pnum);
        SPValidPos(2)=uint8(81)+t_index-t_pnum;
        if SPValidPos(2)>80
            SPValidPos(2)=SPValidPos(2)-80;
        end
        if (SPValidPos(2)>=LM_OTLSPPos&&t_index>=LM_OTLSPPos)||(SPValidPos(2)<LM_OTLSPPos&&t_index<LM_OTLSPPos)
            for i=t_index:-1:SPValidPos(2)
                t_error=(LM_OTLDyVect(i)-t_mean)^2;
                t_sumerry=t_sumerry+t_error;
            end
        else
            for i=1:t_index
                t_error=(LM_OTLDyVect(i)-t_mean)^2;
                t_sumerry=t_sumerry+t_error;
            end
            for i=80:-1:SPValidPos(2)
                t_error=(LM_OTLDyVect(i)-t_mean)^2;
                t_sumerry=t_sumerry+t_error;
            end
        end
        if sqrt(t_sumerry/single(t_pnum))<=P_LM_OTLTrajStdThre
           Offset(2)=t_mean;
           Flg(2)=uint8(1);
           TpValidNum(2)=t_pnum;
        end           
    end
end
%%第三段前车道线取点
t_pnum=uint8(0);
t_sumy=single(0);
t_sumerry=single(0);
t_index=uint8(0);
if LM_OTLBufValidInfo(3)~=0
    if LM_OTLEPPos>=LM_OTLSPPos
        for i=LM_OTLSPPos:LM_OTLEPPos
            if LM_OTLDxVect(i)>LM_FntPath2Dis&&LM_OTLDxVect(i)<=LM_FntPath3Dis
                t_pnum=t_pnum+uint8(1);
                t_index=i;
                t_sumy=t_sumy+LM_OTLDyVect(i);
            end
        end
        SPValidPos(3)=t_index-t_pnum+1;
        t_mean=t_sumy/single(t_pnum);
        for i=t_index:-1:SPValidPos(3)
            t_error=(LM_OTLDyVect(i)-t_mean)^2;
            t_sumerry=t_sumerry+t_error;
        end
        if sqrt(t_sumerry/single(t_pnum))<=P_LM_OTLTrajStdThre
           Offset(3)=t_mean;
           Flg(3)=uint8(1);
           TpValidNum(3)=t_pnum;
        end
    elseif LM_OTLEPPos<LM_OTLSPPos
        for i=LM_OTLSPPos:80
            if LM_OTLDxVect(i)>LM_FntPath2Dis&&LM_OTLDxVect(i)<=LM_FntPath3Dis
                t_pnum=t_pnum+uint8(1);
                t_index=i;
                t_sumy=t_sumy+LM_OTLDyVect(i);
            end
        end
        for i=1:LM_OTLEPPos 
            if LM_OTLDxVect(i)>LM_FntPath2Dis&&LM_OTLDxVect(i)<=LM_FntPath3Dis
                t_pnum=t_pnum+uint8(1);
                t_index=i;
                t_sumy=t_sumy+LM_OTLDyVect(i);
            end
        end
        t_mean=t_sumy/single(t_pnum);
        SPValidPos(3)=uint8(81)+t_index-t_pnum;
        if SPValidPos(3)>80
            SPValidPos(3)=SPValidPos(3)-80;
        end
        if (SPValidPos(3)>=LM_OTLSPPos&&t_index>=LM_OTLSPPos)||(SPValidPos(3)<LM_OTLSPPos&&t_index<LM_OTLSPPos)
            for i=t_index:-1:SPValidPos(3)
                t_error=(LM_OTLDyVect(i)-t_mean)^2;
                t_sumerry=t_sumerry+t_error;
            end
        else
            for i=1:t_index
                t_error=(LM_OTLDyVect(i)-t_mean)^2;
                t_sumerry=t_sumerry+t_error;
            end
            for i=80:-1:SPValidPos(3)
                t_error=(LM_OTLDyVect(i)-t_mean)^2;
                t_sumerry=t_sumerry+t_error;
            end
        end
        if sqrt(t_sumerry/single(t_pnum))<=P_LM_OTLTrajStdThre
           Offset(3)=t_mean;
           Flg(3)=uint8(1);
           TpValidNum(3)=t_pnum;
        end           
    end
end
end

== matlab function PubIfDecisionLM_MDL/Subsystem2/LM_OTL/LM_OTL_MovObjTrajFit/LM_OTL_BufTPAssess/LM_OTL_BufTrajEva/Subsystem1/MATLAB Function1 ==
  data: Offset output; Flg output; LM_OTLBufValidInfo input; LM_OTLDxVect input; LM_OTLDyVect input; LM_OTLSPPos input; LM_OTLEPPos input; LM_FntPath1Dis input; LM_FntPath2Dis input; LM_FntPath3Dis input; TpValidNum output; SPValidPos output; P_LM_OTLTrajStdThre input
function [Offset,Flg,TpValidNum,SPValidPos] = fcn(LM_OTLBufValidInfo,LM_OTLDxVect,LM_OTLDyVect,LM_OTLSPPos,LM_OTLEPPos,LM_FntPath1Dis,LM_FntPath2Dis,LM_FntPath3Dis, P_LM_OTLTrajStdThre)


%%第一段前车道线取点
Offset=single(zeros(3,1));
Flg=uint8(zeros(3,1));
TpValidNum=uint8(zeros(3,1));
SPValidPos=uint8(zeros(3,1));
t_pnum=uint8(0);
t_sumy=single(0);
t_sumerry=single(0);
t_index=uint8(0);
if LM_OTLBufValidInfo(1)~=0
    if LM_OTLEPPos>=LM_OTLSPPos
        for i=LM_OTLSPPos:LM_OTLEPPos
            if LM_OTLDxVect(i)>0&&LM_OTLDxVect(i)<=LM_FntPath1Dis
                t_pnum=t_pnum+uint8(1);
                t_index=i;
                t_sumy=t_sumy+LM_OTLDyVect(i);
            end
        end
        t_mean=t_sumy/single(t_pnum);
        SPValidPos(1)=t_index-t_pnum+uint8(1);
        for i=t_index:-1:SPValidPos(1)
            t_error=(LM_OTLDyVect(i)-t_mean)^2;
            t_sumerry=t_sumerry+t_error;
        end
        if sqrt(t_sumerry/single(t_pnum))<=P_LM_OTLTrajStdThre
           Offset(1)=t_mean;
           Flg(1)=uint8(1);
           TpValidNum(1)=t_pnum;
        end
    elseif LM_OTLEPPos<LM_OTLSPPos
        for i=LM_OTLSPPos:80
            if LM_OTLDxVect(i)>0&&LM_OTLDxVect(i)<=LM_FntPath1Dis
                t_pnum=t_pnum+uint8(1);
                t_index=i;
                t_sumy=t_sumy+LM_OTLDyVect(i);
            end
        end
        for i=1:LM_OTLEPPos 
            if LM_OTLDxVect(i)>0&&LM_OTLDxVect(i)<=LM_FntPath1Dis
                t_pnum=t_pnum+uint8(1);
                t_index=i;
                t_sumy=t_sumy+LM_OTLDyVect(i);
            end
        end
        SPValidPos(1)=uint8(81)+t_index-t_pnum;
        t_mean=t_sumy/single(t_pnum);
        if SPValidPos(1)>80
            SPValidPos(1)=SPValidPos(1)-80;
        end
        if (SPValidPos(1)>=LM_OTLSPPos&&t_index>=LM_OTLSPPos)||(SPValidPos(1)<LM_OTLSPPos&&t_index<LM_OTLSPPos)
            for i=t_index:-1:SPValidPos(1)
                t_error=(LM_OTLDyVect(i)-t_mean)^2;
                t_sumerry=t_sumerry+t_error;
            end
        else
            for i=1:t_index
                t_error=(LM_OTLDyVect(i)-t_mean)^2;
                t_sumerry=t_sumerry+t_error;
            end
            for i=80:-1:SPValidPos(1)
                 t_error=(LM_OTLDyVect(i)-t_mean)^2;
                t_sumerry=t_sumerry+t_error;
            end
        end
        if sqrt(t_sumerry/single(t_pnum))<=P_LM_OTLTrajStdThre
           Offset(1)=t_mean;
           Flg(1)=uint8(1);
           TpValidNum(1)=t_pnum;
        end           
    end
end
%%第二段前车道线取点
t_pnum=uint8(0);
t_sumy=single(0);
t_sumerry=single(0);
t_index=uint8(0);
if LM_OTLBufValidInfo(2)~=0
    if LM_OTLEPPos>=LM_OTLSPPos
        for i=LM_OTLSPPos:LM_OTLEPPos
            if LM_OTLDxVect(i)>LM_FntPath1Dis&&LM_OTLDxVect(i)<=LM_FntPath2Dis
                t_pnum=t_pnum+uint8(1);
                t_index=i;
                t_sumy=t_sumy+LM_OTLDyVect(i);
            end
        end
        t_mean=t_sumy/single(t_pnum);
        SPValidPos(2)=t_index-t_pnum+uint8(1);
        for i=t_index:-1:SPValidPos(2)
            t_error=(LM_OTLDyVect(i)-t_mean)^2;
            t_sumerry=t_sumerry+t_error;
        end
        if sqrt(t_sumerry/single(t_pnum))<=P_LM_OTLTrajStdThre
           Offset(2)=t_mean;
           Flg(2)=uint8(1);
           TpValidNum(2)=t_pnum;
        end
    elseif LM_OTLEPPos<LM_OTLSPPos
        for i=LM_OTLSPPos:80
            if LM_OTLDxVect(i)>LM_FntPath1Dis&&LM_OTLDxVect(i)<=LM_FntPath2Dis
                t_pnum=t_pnum+uint8(1);
                t_index=i;
                t_sumy=t_sumy+LM_OTLDyVect(i);
            end
        end
        for i=1:LM_OTLEPPos 
            if LM_OTLDxVect(i)>LM_FntPath1Dis&&LM_OTLDxVect(i)<=LM_FntPath2Dis
                t_pnum=t_pnum+uint8(1);
                t_index=i;
                t_sumy=t_sumy+LM_OTLDyVect(i);
            end
        end
        t_mean=t_sumy/single(t_pnum);
        SPValidPos(2)=uint8(81)+t_index-t_pnum;
        if SPValidPos(2)>80
            SPValidPos(2)=SPValidPos(2)-80;
        end
        if (SPValidPos(2)>=LM_OTLSPPos&&t_index>=LM_OTLSPPos)||(SPValidPos(2)<LM_OTLSPPos&&t_index<LM_OTLSPPos)
            for i=t_index:-1:SPValidPos(2)
                t_error=(LM_OTLDyVect(i)-t_mean)^2;
                t_sumerry=t_sumerry+t_error;
            end
        else
            for i=1:t_index
                t_error=(LM_OTLDyVect(i)-t_mean)^2;
                t_sumerry=t_sumerry+t_error;
            end
            for i=80:-1:SPValidPos(2)
                t_error=(LM_OTLDyVect(i)-t_mean)^2;
                t_sumerry=t_sumerry+t_error;
            end
        end
        if sqrt(t_sumerry/single(t_pnum))<=P_LM_OTLTrajStdThre
           Offset(2)=t_mean;
           Flg(2)=uint8(1);
           TpValidNum(2)=t_pnum;
        end           
    end
end
%%第三段前车道线取点
t_pnum=uint8(0);
t_sumy=single(0);
t_sumerry=single(0);
t_index=uint8(0);
if LM_OTLBufValidInfo(3)~=0
    if LM_OTLEPPos>=LM_OTLSPPos
        for i=LM_OTLSPPos:LM_OTLEPPos
            if LM_OTLDxVect(i)>LM_FntPath2Dis&&LM_OTLDxVect(i)<=LM_FntPath3Dis
                t_pnum=t_pnum+uint8(1);
                t_index=i;
                t_sumy=t_sumy+LM_OTLDyVect(i);
            end
        end
        SPValidPos(3)=t_index-t_pnum+1;
        t_mean=t_sumy/single(t_pnum);
        for i=t_index:-1:SPValidPos(3)
            t_error=(LM_OTLDyVect(i)-t_mean)^2;
            t_sumerry=t_sumerry+t_error;
        end
        if sqrt(t_sumerry/single(t_pnum))<=P_LM_OTLTrajStdThre
           Offset(3)=t_mean;
           Flg(3)=uint8(1);
           TpValidNum(3)=t_pnum;
        end
    elseif LM_OTLEPPos<LM_OTLSPPos
        for i=LM_OTLSPPos:80
            if LM_OTLDxVect(i)>LM_FntPath2Dis&&LM_OTLDxVect(i)<=LM_FntPath3Dis
                t_pnum=t_pnum+uint8(1);
                t_index=i;
                t_sumy=t_sumy+LM_OTLDyVect(i);
            end
        end
        for i=1:LM_OTLEPPos 
            if LM_OTLDxVect(i)>LM_FntPath2Dis&&LM_OTLDxVect(i)<=LM_FntPath3Dis
                t_pnum=t_pnum+uint8(1);
                t_index=i;
                t_sumy=t_sumy+LM_OTLDyVect(i);
            end
        end
        t_mean=t_sumy/single(t_pnum);
        SPValidPos(3)=uint8(81)+t_index-t_pnum;
        if SPValidPos(3)>80
            SPValidPos(3)=SPValidPos(3)-80;
        end
        if (SPValidPos(3)>=LM_OTLSPPos&&t_index>=LM_OTLSPPos)||(SPValidPos(3)<LM_OTLSPPos&&t_index<LM_OTLSPPos)
            for i=t_index:-1:SPValidPos(3)
                t_error=(LM_OTLDyVect(i)-t_mean)^2;
                t_sumerry=t_sumerry+t_error;
            end
        else
            for i=1:t_index
                t_error=(LM_OTLDyVect(i)-t_mean)^2;
                t_sumerry=t_sumerry+t_error;
            end
            for i=80:-1:SPValidPos(3)
                t_error=(LM_OTLDyVect(i)-t_mean)^2;
                t_sumerry=t_sumerry+t_error;
            end
        end
        if sqrt(t_sumerry/single(t_pnum))<=P_LM_OTLTrajStdThre
           Offset(3)=t_mean;
           Flg(3)=uint8(1);
           TpValidNum(3)=t_pnum;
        end           
    end
end
end

== matlab function PubIfDecisionLM_MDL/Subsystem2/LM_OTL/LM_OTL_MovObjTrajFit/LM_OTL_BufTPAssess/LM_OTL_BufTrajEva/Subsystem10/MATLAB Function1 ==
  data: Offset output; Flg output; LM_OTLBufValidInfo input; LM_OTLDxVect input; LM_OTLDyVect input; LM_OTLSPPos input; LM_OTLEPPos input; LM_FntPath1Dis input; LM_FntPath2Dis input; LM_FntPath3Dis input; TpValidNum output; SPValidPos output; P_LM_OTLTrajStdThre input
function [Offset,Flg,TpValidNum,SPValidPos] = fcn(LM_OTLBufValidInfo,LM_OTLDxVect,LM_OTLDyVect,LM_OTLSPPos,LM_OTLEPPos,LM_FntPath1Dis,LM_FntPath2Dis,LM_FntPath3Dis, P_LM_OTLTrajStdThre)


%%第一段前车道线取点
Offset=single(zeros(3,1));
Flg=uint8(zeros(3,1));
TpValidNum=uint8(zeros(3,1));
SPValidPos=uint8(zeros(3,1));
t_pnum=uint8(0);
t_sumy=single(0);
t_sumerry=single(0);
t_index=uint8(0);
if LM_OTLBufValidInfo(1)~=0
    if LM_OTLEPPos>=LM_OTLSPPos
        for i=LM_OTLSPPos:LM_OTLEPPos
            if LM_OTLDxVect(i)>0&&LM_OTLDxVect(i)<=LM_FntPath1Dis
                t_pnum=t_pnum+uint8(1);
                t_index=i;
                t_sumy=t_sumy+LM_OTLDyVect(i);
            end
        end
        t_mean=t_sumy/single(t_pnum);
        SPValidPos(1)=t_index-t_pnum+uint8(1);
        for i=t_index:-1:SPValidPos(1)
            t_error=(LM_OTLDyVect(i)-t_mean)^2;
            t_sumerry=t_sumerry+t_error;
        end
        if sqrt(t_sumerry/single(t_pnum))<=P_LM_OTLTrajStdThre
           Offset(1)=t_mean;
           Flg(1)=uint8(1);
           TpValidNum(1)=t_pnum;
        end
    elseif LM_OTLEPPos<LM_OTLSPPos
        for i=LM_OTLSPPos:80
            if LM_OTLDxVect(i)>0&&LM_OTLDxVect(i)<=LM_FntPath1Dis
                t_pnum=t_pnum+uint8(1);
                t_index=i;
                t_sumy=t_sumy+LM_OTLDyVect(i);
            end
        end
        for i=1:LM_OTLEPPos 
            if LM_OTLDxVect(i)>0&&LM_OTLDxVect(i)<=LM_FntPath1Dis
                t_pnum=t_pnum+uint8(1);
                t_index=i;
                t_sumy=t_sumy+LM_OTLDyVect(i);
            end
        end
        SPValidPos(1)=uint8(81)+t_index-t_pnum;
        t_mean=t_sumy/single(t_pnum);
        if SPValidPos(1)>80
            SPValidPos(1)=SPValidPos(1)-80;
        end
        if (SPValidPos(1)>=LM_OTLSPPos&&t_index>=LM_OTLSPPos)||(SPValidPos(1)<LM_OTLSPPos&&t_index<LM_OTLSPPos)
            for i=t_index:-1:SPValidPos(1)
                t_error=(LM_OTLDyVect(i)-t_mean)^2;
                t_sumerry=t_sumerry+t_error;
            end
        else
            for i=1:t_index
                t_error=(LM_OTLDyVect(i)-t_mean)^2;
                t_sumerry=t_sumerry+t_error;
            end
            for i=80:-1:SPValidPos(1)
                 t_error=(LM_OTLDyVect(i)-t_mean)^2;
                t_sumerry=t_sumerry+t_error;
            end
        end
        if sqrt(t_sumerry/single(t_pnum))<=P_LM_OTLTrajStdThre
           Offset(1)=t_mean;
           Flg(1)=uint8(1);
           TpValidNum(1)=t_pnum;
        end           
    end
end
%%第二段前车道线取点
t_pnum=uint8(0);
t_sumy=single(0);
t_sumerry=single(0);
t_index=uint8(0);
if LM_OTLBufValidInfo(2)~=0
    if LM_OTLEPPos>=LM_OTLSPPos
        for i=LM_OTLSPPos:LM_OTLEPPos
            if LM_OTLDxVect(i)>LM_FntPath1Dis&&LM_OTLDxVect(i)<=LM_FntPath2Dis
                t_pnum=t_pnum+uint8(1);
                t_index=i;
                t_sumy=t_sumy+LM_OTLDyVect(i);
            end
        end
        t_mean=t_sumy/single(t_pnum);
        SPValidPos(2)=t_index-t_pnum+uint8(1);
        for i=t_index:-1:SPValidPos(2)
            t_error=(LM_OTLDyVect(i)-t_mean)^2;
            t_sumerry=t_sumerry+t_error;
        end
        if sqrt(t_sumerry/single(t_pnum))<=P_LM_OTLTrajStdThre
           Offset(2)=t_mean;
           Flg(2)=uint8(1);
           TpValidNum(2)=t_pnum;
        end
    elseif LM_OTLEPPos<LM_OTLSPPos
        for i=LM_OTLSPPos:80
            if LM_OTLDxVect(i)>LM_FntPath1Dis&&LM_OTLDxVect(i)<=LM_FntPath2Dis
                t_pnum=t_pnum+uint8(1);
                t_index=i;
                t_sumy=t_sumy+LM_OTLDyVect(i);
            end
        end
        for i=1:LM_OTLEPPos 
            if LM_OTLDxVect(i)>LM_FntPath1Dis&&LM_OTLDxVect(i)<=LM_FntPath2Dis
                t_pnum=t_pnum+uint8(1);
                t_index=i;
                t_sumy=t_sumy+LM_OTLDyVect(i);
            end
        end
        t_mean=t_sumy/single(t_pnum);
        SPValidPos(2)=uint8(81)+t_index-t_pnum;
        if SPValidPos(2)>80
            SPValidPos(2)=SPValidPos(2)-80;
        end
        if (SPValidPos(2)>=LM_OTLSPPos&&t_index>=LM_OTLSPPos)||(SPValidPos(2)<LM_OTLSPPos&&t_index<LM_OTLSPPos)
            for i=t_index:-1:SPValidPos(2)
                t_error=(LM_OTLDyVect(i)-t_mean)^2;
                t_sumerry=t_sumerry+t_error;
            end
        else
            for i=1:t_index
                t_error=(LM_OTLDyVect(i)-t_mean)^2;
                t_sumerry=t_sumerry+t_error;
            end
            for i=80:-1:SPValidPos(2)
                t_error=(LM_OTLDyVect(i)-t_mean)^2;
                t_sumerry=t_sumerry+t_error;
            end
        end
        if sqrt(t_sumerry/single(t_pnum))<=P_LM_OTLTrajStdThre
           Offset(2)=t_mean;
           Flg(2)=uint8(1);
           TpValidNum(2)=t_pnum;
        end           
    end
end
%%第三段前车道线取点
t_pnum=uint8(0);
t_sumy=single(0);
t_sumerry=single(0);
t_index=uint8(0);
if LM_OTLBufValidInfo(3)~=0
    if LM_OTLEPPos>=LM_OTLSPPos
        for i=LM_OTLSPPos:LM_OTLEPPos
            if LM_OTLDxVect(i)>LM_FntPath2Dis&&LM_OTLDxVect(i)<=LM_FntPath3Dis
                t_pnum=t_pnum+uint8(1);
                t_index=i;
                t_sumy=t_sumy+LM_OTLDyVect(i);
            end
        end
        SPValidPos(3)=t_index-t_pnum+1;
        t_mean=t_sumy/single(t_pnum);
        for i=t_index:-1:SPValidPos(3)
            t_error=(LM_OTLDyVect(i)-t_mean)^2;
            t_sumerry=t_sumerry+t_error;
        end
        if sqrt(t_sumerry/single(t_pnum))<=P_LM_OTLTrajStdThre
           Offset(3)=t_mean;
           Flg(3)=uint8(1);
           TpValidNum(3)=t_pnum;
        end
    elseif LM_OTLEPPos<LM_OTLSPPos
        for i=LM_OTLSPPos:80
            if LM_OTLDxVect(i)>LM_FntPath2Dis&&LM_OTLDxVect(i)<=LM_FntPath3Dis
                t_pnum=t_pnum+uint8(1);
                t_index=i;
                t_sumy=t_sumy+LM_OTLDyVect(i);
            end
        end
        for i=1:LM_OTLEPPos 
            if LM_OTLDxVect(i)>LM_FntPath2Dis&&LM_OTLDxVect(i)<=LM_FntPath3Dis
                t_pnum=t_pnum+uint8(1);
                t_index=i;
                t_sumy=t_sumy+LM_OTLDyVect(i);
            end
        end
        t_mean=t_sumy/single(t_pnum);
        SPValidPos(3)=uint8(81)+t_index-t_pnum;
        if SPValidPos(3)>80
            SPValidPos(3)=SPValidPos(3)-80;
        end
        if (SPValidPos(3)>=LM_OTLSPPos&&t_index>=LM_OTLSPPos)||(SPValidPos(3)<LM_OTLSPPos&&t_index<LM_OTLSPPos)
            for i=t_index:-1:SPValidPos(3)
                t_error=(LM_OTLDyVect(i)-t_mean)^2;
                t_sumerry=t_sumerry+t_error;
            end
        else
            for i=1:t_index
                t_error=(LM_OTLDyVect(i)-t_mean)^2;
                t_sumerry=t_sumerry+t_error;
            end
            for i=80:-1:SPValidPos(3)
                t_error=(LM_OTLDyVect(i)-t_mean)^2;
                t_sumerry=t_sumerry+t_error;
            end
        end
        if sqrt(t_sumerry/single(t_pnum))<=P_LM_OTLTrajStdThre
           Offset(3)=t_mean;
           Flg(3)=uint8(1);
           TpValidNum(3)=t_pnum;
        end           
    end
end
end
